simulink model "firstTry"  (R2013b)
settings: Solver=ode45  StartTime=0  StopTime=100  RelTol=1e-3
libraries: simulink_extras x2
settings Model: Creator=Maksimus  LastModifiedBy=Maksimus

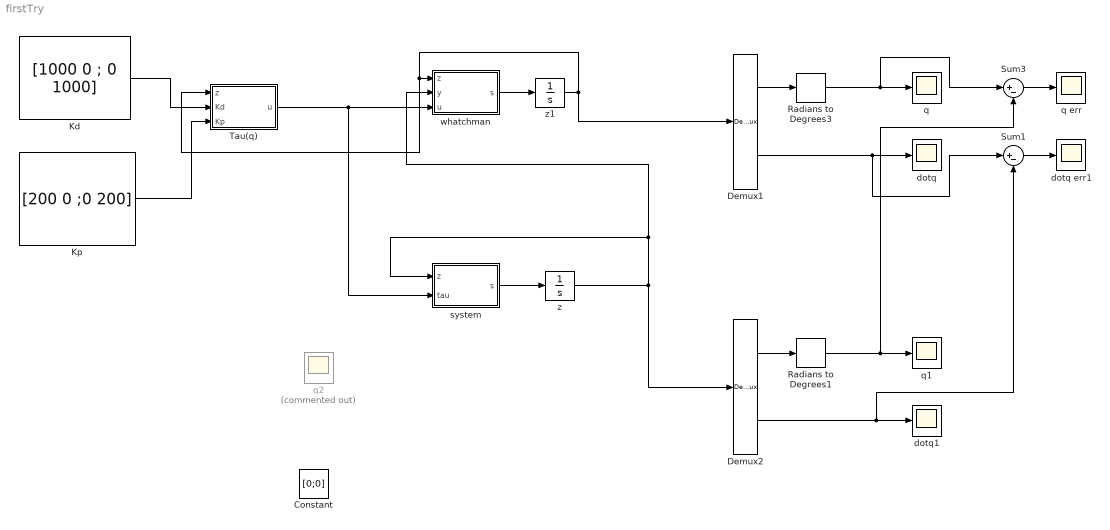
== system firstTry ==
  Constant : Constant  Value=[0;0]
  Demux1 : Demux  Outputs=2
  Demux2 : Demux  Outputs=2
  Kd : Constant  Value=[1000 0 ; 0 1000]
  "Kp " : Constant  Value=[200 0 ;0 200]
  Radians to Degrees1 : simulink_extras/Transformations/Radians to Degrees
  Radians to Degrees3 : simulink_extras/Transformations/Radians to Degrees
  Sum1 : Sum  Inputs=|+-
  Sum3 : Sum  Inputs=|+-
  Tau(q) : MATLAB Function  TreatAsAtomicUnit=on
  dotq : Scope
      settings: YMin=-0.000325  YMax=-2.5e-05
  dotq err1 : Scope
      settings: YMin=-0.000325  YMax=-2.5e-05  SaveName=ScopeData2
  dotq1 : Scope
      settings: YMin=-0.000325  YMax=-2.5e-05  SaveName=ScopeData3
  q : Scope
      settings: YMin=-0.000325  YMax=-2.5e-05  SaveName=ScopeData5
  q err : Scope
      settings: YMin=-4.5e+06  YMax=2.5e+06
  q1 : Scope
      settings: YMin=-2.5e+06  YMax=1.5e+06  SaveName=ScopeData4
  q2 : Scope  Commented=on
      settings: YMin=-2.5e+06  YMax=1.5e+06  SaveName=ScopeData6
  system : MATLAB Function  TreatAsAtomicUnit=on
  "whatchman " : MATLAB Function  TreatAsAtomicUnit=on
  z : Integrator  InitialCondition=[-pi/2;0;pi/180;0]  IgnoreLimit=on
  z1 : Integrator  InitialCondition=[-pi/2;0; 0;0]  IgnoreLimit=on
  wires:
  "whatchman "/1(s) -> z1/1
  Kd/1 -> Tau(q)/2(Kd)
  "Kp "/1 -> Tau(q)/3(Kp)
  system/1(s) -> z/1
  Tau(q)/1(u) -> system/2(tau), "whatchman "/3(u)
  Radians to Degrees3/1 -> Sum3/1, q/1
  z1/1 -> Tau(q)/1(z), "whatchman "/1(z), Demux1/1
  Demux1/1 -> Radians to Degrees3/1
  Demux1/2 -> Sum1/1, dotq/1
  Sum3/1 -> q err/1
  Sum1/1 -> dotq err1/1
  Radians to Degrees1/1 -> Sum3/2, q1/1
  Demux2/1 -> Radians to Degrees1/1
  Demux2/2 -> Sum1/2, dotq1/1
  z/1 -> system/1(z), "whatchman "/2(y), Demux2/1

== matlab function firstTry/whatchman  ==
  data: z input; y input; s output; u input
function s = fcn(z,y,u)
linA = [  0, 0, 1, 0;
    0, 0, 0, 1;
    -26500/2959, +25000/2959, 0, 0;
    +25000/2959,  -51500/2959, 0, 0];

linB = [          0,          0;
        0,          0;
        2575/2959, -3825/2959;
 -3825/2959,  6400/2959];
Gg=[-70  30 ; 32  60;   4  -9;  95  -14];
%[-11, 22; -11, 1000; -10, -120; -11,-11]*1000;
%[-11, 0; -11, 11; -10, -120; -11,-11] * 1000;
CC = [ 1 0 0 0;
      0 1  0 0];

 y = [y(1);y(2)];
 CC = [0 0 0 0; 0 0 0 0];
s = (double(linA) + Gg * CC)* z - Gg*y+linB * u;

== matlab function firstTry/Tau(q) ==
  data: z input; u output; Kd input; Kp input
function u= fcn(z, Kd, Kp)
qn = [-pi/2;0];

m1 = 1;
m2 = 1;
lc1 = 1;
lc2 = 2;
I1 = 0.12;
I2 = 0.12;
l1 = 1;
l2 = 1;
g=10;

m = [m1;m2];
lc = [lc1;lc2];
I = [I1;I2];
l = [l1;l2];
theta = [m(1)*lc(1)^2 + m(2)*l(1)^2 + I(1); m(2) * lc(2)^2 + I(2); m(2)*l(1)*lc(2); m(1)*lc(1) + m(2)*l(1); m(2)*lc(2)]; 
%is symmetrie, positive definite for all q

%H(q) - 2C(q, dotq) is a skew-syrnmetric matrix

H = [theta(1) + theta(2) + 2 * theta(3)*cos(z(2)), theta(2) + theta(3) * cos(z(2));
    theta(2) + theta(3) * cos(z(2)), theta(2)]; 

G = [ theta(4) * g * cos(z(1)) + theta(5) * g * cos(z(1) + z(2)); theta(5) * g * cos(z(1) + z(2))];
G = [0;0];

qp  = [z(1);z(2)] - qn;
tau = -Kd * [z(3);z(4)] - Kp*qp + G;

u =tau;

== matlab function firstTry/system ==
  data: z input; s output; tau input
function s = fcn(z,tau)
%global linA linB linConst
%s = linA * z + linB * u + linConst;
m1 = 1;
m2 = 1;
lc1 = 1;
lc2 = 2;
I1 = 0.12;
I2 = 0.12;
l1 = 1;
l2 = 1;
g=10;

m = [m1;m2];
lc = [lc1;lc2];
I = [I1;I2];
l = [l1;l2];
dotq = z(3:4);
q = z(1:2);
theta = [m(1)*lc(1)^2 + m(2)*l(1)^2 + I(1); m(2) * lc(2)^2 + I(2); m(2)*l(1)*lc(2); m(1)*lc(1) + m(2)*l(1); m(2)*lc(2)]; 

H = [theta(1) + theta(2) + 2 * theta(3)*cos(q(2)), theta(2) + theta(3) * cos(q(2));
    theta(2) + theta(3) * cos(q(2)), theta(2)]; %is symmetrie, positive definite for all q

%H(q) - 2C(q, dotq) is a skew-syrnmetric matrix

C = [-theta(3) * sin(q(2)) * dotq(2), -theta(3) * sin(q(2)) * dotq(2) - theta(3) * sin(q(2)) * dotq(1);
    theta(3) * sin(q(2)) * dotq(1), 0];

G = [ theta(4) * g * cos(q(1)) + theta(5) * g * cos(q(1) + q(2)); theta(5) * g * cos(q(1) + q(2))]; %nonhorizontal robotarm

InvH = H^(-1);
InvHC = InvH * C;
InvHG = InvH * G;
tmpsys = - InvHC * dotq - InvHG + InvH*tau;
sys = [dotq;tmpsys];

s = sys;
